simulink model "check_Transmission"  (R2018b)
settings: configuration reference "Physics" (kept outside this file)
model workspace (MAT data in the model file):
  veh_param = Simulink.Parameter
  veh_param.Value.cLiftF = 0
  veh_param.Value.cLiftR = 0
  veh_param.Value.CoGx_m = 0
  veh_param.Value.CoGy_m = 0
  veh_param.Value.CoGz_m = 0
  veh_param.Value.cDrag = 0
  veh_param.Value.Aref_m2 = 0
  veh_param.Value.Gearratio = 0
  veh_param.Value.Wheelbase_m = 0
  veh_param.Value.PacLatF = [0 0 0 0 0]
  veh_param.Value.PacLongF = [0 0 0 0 0]
  veh_param.Value.PacLatR = [0 0 0 0 0]
  veh_param.Value.PacLongR = [0 0 0 0 0]
  veh_param.Value.cRollFriction_Npmps = 0
  veh_param.Value.MaxRollFriction_N = 0
  veh_param.Value.T_YawRate_s = 0
  veh_param.Value.T_LatVel_s = 0
  veh_param.Value.TrackWidthF_m = 0
  veh_param.Value.TrackWidthR_m = 0
  veh_param.Value.TireRadiusF_m = 0
  veh_param.Value.TireRadiusR_m = 0
  veh_param.Value.VehicleInertia_kgm2 = 0
  veh_param.Value.WheelInertiaF_kgm2 = 0
  veh_param.Value.WheelInertiaR_kgm2 = 0
  veh_param.Value.VehicleMass_kg = 0
  veh_param.Value.switchModelBlend_mps = 0
  veh_param.Value.PTLimitLowVel_N = 0
  veh_param.Value.switchModelVel_mps = 0
  veh_param.Value.T_Tire_s = 0
  veh_param.DataType = 'struct'
  veh_param.Dimensions = [1 1]
  x0_positionstates = Simulink.Parameter
  x0_positionstates.Value = [0 0 0]
  x0_positionstates.DataType = 'auto'
  x0_positionstates.Dimensions = [1 3]
undefined symbols (not defined in the file): POWTR__ENGINE__n_lb_rpm__1, POWTR__ENGINE__n_lb_rpm__2, POWTR__ENGINE__n_lb_rpm__3, POWTR__ENGINE__n_lb_rpm__4, POWTR__ENGINE__n_lb_rpm__5, POWTR__ENGINE__n_lb_rpm__6, POWTR__ENGINE__n_lb_rpm__7, POWTR__TRANSMISSION__gear__1, POWTR__TRANSMISSION__gear__2, POWTR__TRANSMISSION__gear__3, POWTR__TRANSMISSION__gear__4, POWTR__TRANSMISSION__gear__5, POWTR__TRANSMISSION__gear__6, POWTR__TRANSMISSION__gear__7, POWTR__TRANSMISSION__gear_efficiency__1, POWTR__TRANSMISSION__gear_efficiency__2, POWTR__TRANSMISSION__gear_efficiency__3, POWTR__TRANSMISSION__gear_efficiency__4, POWTR__TRANSMISSION__gear_efficiency__5, POWTR__TRANSMISSION__gear_efficiency__6, POWTR__TRANSMISSION__gear_efficiency__7, POWTR__TRANSMISSION__gear_ratio__1, POWTR__TRANSMISSION__gear_ratio__2, POWTR__TRANSMISSION__gear_ratio__3, POWTR__TRANSMISSION__gear_ratio__4, POWTR__TRANSMISSION__gear_ratio__5, POWTR__TRANSMISSION__gear_ratio__6, POWTR__TRANSMISSION__gear_ratio__7
settings Model: DataDictionary=vehicleparameters_vehdynsim.sldd  OrderedModelArguments=off  Creator=wischnewski  LastModifiedBy=ga25xiw

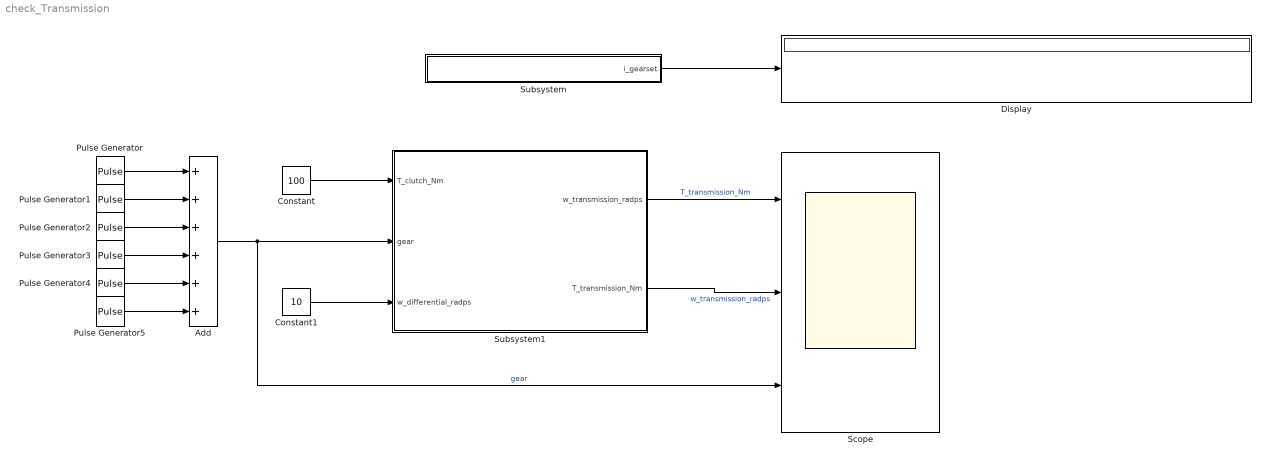
== system check_Transmission ==
  Add : Sum  Inputs=++++++
  Constant : Constant  Value=100
  Constant1 : Constant  Value=10
  Display : Display
  Pulse Generator : DiscretePulseGenerator  PulseType=Time based  Period=10  PulseWidth=90  PhaseDelay=2
  Pulse Generator1 : DiscretePulseGenerator  PulseType=Time based  Period=10  PulseWidth=90  PhaseDelay=3
  Pulse Generator2 : DiscretePulseGenerator  PulseType=Time based  Period=10  PulseWidth=90  PhaseDelay=4
  Pulse Generator3 : DiscretePulseGenerator  PulseType=Time based  Period=10  PulseWidth=90  PhaseDelay=5
  Pulse Generator4 : DiscretePulseGenerator  PulseType=Time based  Period=10  PulseWidth=90  PhaseDelay=6
  Pulse Generator5 : DiscretePulseGenerator  PulseType=Time based  Period=10  PulseWidth=90  PhaseDelay=7
  Scope : Scope  NumInputPorts=3
  Subsystem : Subsystem
  Subsystem1 : Subsystem
  wires:
  Subsystem1/1(w_transmission_radps) -> Scope/1  "T_transmission_Nm"
  Subsystem1/2(T_transmission_Nm) -> Scope/2  "w_transmission_radps"
  Constant/1 -> Subsystem1/1(T_clutch_Nm)
  Pulse Generator/1 -> Add/1
  Pulse Generator1/1 -> Add/2
  Pulse Generator2/1 -> Add/3
  Pulse Generator3/1 -> Add/4
  Pulse Generator4/1 -> Add/5
  Pulse Generator5/1 -> Add/6
  Add/1 -> Subsystem1/2(gear), Scope/3  "gear"
  Constant1/1 -> Subsystem1/3(w_differential_radps)
  Subsystem/1(i_gearset) -> Display/1

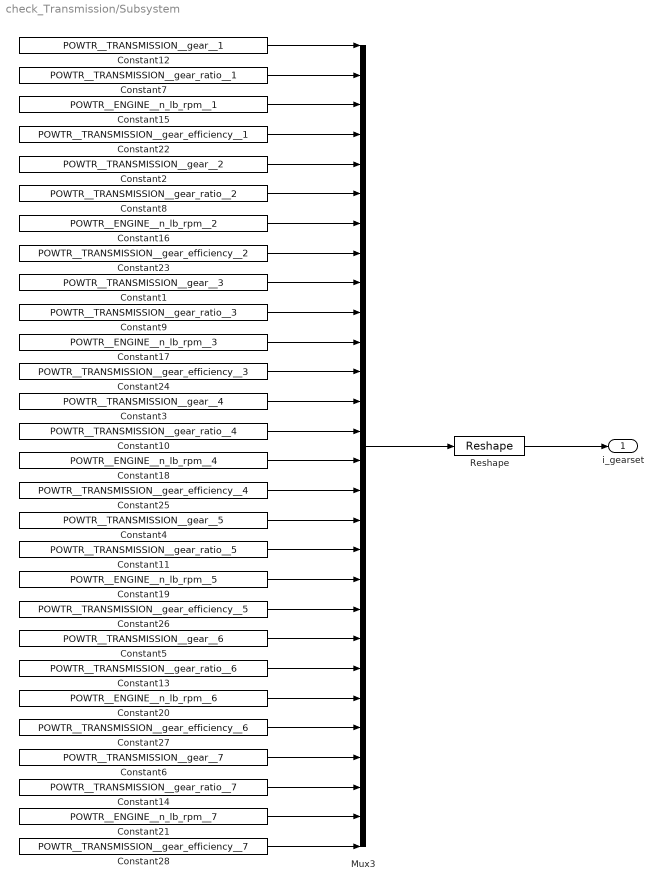
== system check_Transmission/Subsystem ==
  Constant1 : Constant  Value=POWTR__TRANSMISSION__gear__3
  Constant10 : Constant  Value=POWTR__TRANSMISSION__gear_ratio__4
  Constant11 : Constant  Value=POWTR__TRANSMISSION__gear_ratio__5
  Constant12 : Constant  Value=POWTR__TRANSMISSION__gear__1
  Constant13 : Constant  Value=POWTR__TRANSMISSION__gear_ratio__6
  Constant14 : Constant  Value=POWTR__TRANSMISSION__gear_ratio__7
  Constant15 : Constant  Value=POWTR__ENGINE__n_lb_rpm__1
  Constant16 : Constant  Value=POWTR__ENGINE__n_lb_rpm__2
  Constant17 : Constant  Value=POWTR__ENGINE__n_lb_rpm__3
  Constant18 : Constant  Value=POWTR__ENGINE__n_lb_rpm__4
  Constant19 : Constant  Value=POWTR__ENGINE__n_lb_rpm__5
  Constant2 : Constant  Value=POWTR__TRANSMISSION__gear__2
  Constant20 : Constant  Value=POWTR__ENGINE__n_lb_rpm__6
  Constant21 : Constant  Value=POWTR__ENGINE__n_lb_rpm__7
  Constant22 : Constant  Value=POWTR__TRANSMISSION__gear_efficiency__1
  Constant23 : Constant  Value=POWTR__TRANSMISSION__gear_efficiency__2
  Constant24 : Constant  Value=POWTR__TRANSMISSION__gear_efficiency__3
  Constant25 : Constant  Value=POWTR__TRANSMISSION__gear_efficiency__4
  Constant26 : Constant  Value=POWTR__TRANSMISSION__gear_efficiency__5
  Constant27 : Constant  Value=POWTR__TRANSMISSION__gear_efficiency__6
  Constant28 : Constant  Value=POWTR__TRANSMISSION__gear_efficiency__7
  Constant3 : Constant  Value=POWTR__TRANSMISSION__gear__4
  Constant4 : Constant  Value=POWTR__TRANSMISSION__gear__5
  Constant5 : Constant  Value=POWTR__TRANSMISSION__gear__6
  Constant6 : Constant  Value=POWTR__TRANSMISSION__gear__7
  Constant7 : Constant  Value=POWTR__TRANSMISSION__gear_ratio__1
  Constant8 : Constant  Value=POWTR__TRANSMISSION__gear_ratio__2
  Constant9 : Constant  Value=POWTR__TRANSMISSION__gear_ratio__3
  Mux3 : Mux  Inputs=28
  Reshape : Reshape  OutputDimensionality=Customize  OutputDimensions=[4,7]
  i_gearset : Outport
  wires:
  Mux3/1 -> Reshape/1
  Constant12/1 -> Mux3/1
  Reshape/1 -> i_gearset/1
  Constant2/1 -> Mux3/5
  Constant1/1 -> Mux3/9
  Constant3/1 -> Mux3/13
  Constant4/1 -> Mux3/17
  Constant5/1 -> Mux3/21
  Constant6/1 -> Mux3/25
  Constant7/1 -> Mux3/2
  Constant8/1 -> Mux3/6
  Constant9/1 -> Mux3/10
  Constant10/1 -> Mux3/14
  Constant11/1 -> Mux3/18
  Constant13/1 -> Mux3/22
  Constant14/1 -> Mux3/26
  Constant15/1 -> Mux3/3
  Constant16/1 -> Mux3/7
  Constant17/1 -> Mux3/11
  Constant18/1 -> Mux3/15
  Constant19/1 -> Mux3/19
  Constant20/1 -> Mux3/23
  Constant21/1 -> Mux3/27
  Constant22/1 -> Mux3/4
  Constant23/1 -> Mux3/8
  Constant24/1 -> Mux3/12
  Constant25/1 -> Mux3/16
  Constant26/1 -> Mux3/20
  Constant27/1 -> Mux3/24
  Constant28/1 -> Mux3/28

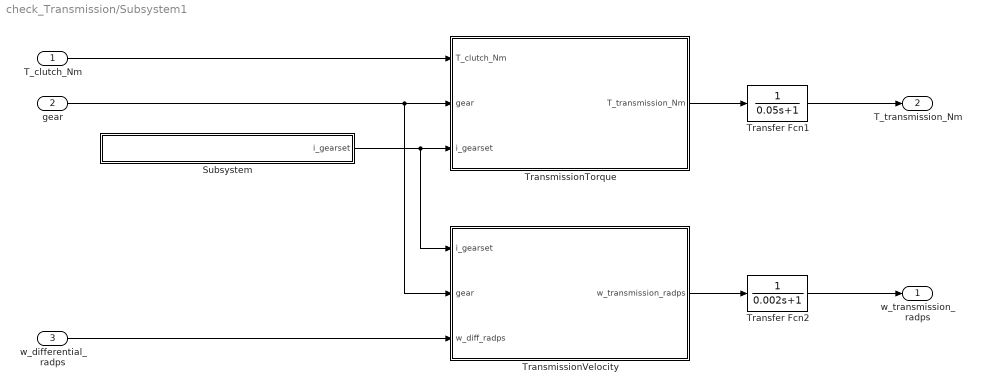
== system check_Transmission/Subsystem1 ==
  T_clutch_Nm : Inport
  gear : Inport  Port=2
  w_differential_radps : Inport  Port=3
  Subsystem : Subsystem
  Transfer Fcn1 : TransferFcn  Denominator=[0.05 1]
  Transfer Fcn2 : TransferFcn  Denominator=[0.002 1]
  TransmissionTorque : MATLAB Function  TreatAsAtomicUnit=on
  TransmissionVelocity : MATLAB Function  TreatAsAtomicUnit=on
  w_transmission_radps : Outport
  T_transmission_Nm : Outport  Port=2
  wires:
  Transfer Fcn1/1 -> T_transmission_Nm/1
  gear/1 -> TransmissionTorque/2(gear), TransmissionVelocity/2(gear)
  Subsystem/1(i_gearset) -> TransmissionTorque/3(i_gearset), TransmissionVelocity/1(i_gearset)
  w_differential_radps/1 -> TransmissionVelocity/3(w_diff_radps)
  Transfer Fcn2/1 -> w_transmission_radps/1
  T_clutch_Nm/1 -> TransmissionTorque/1(T_clutch_Nm)
  TransmissionVelocity/1(w_transmission_radps) -> Transfer Fcn2/1
  TransmissionTorque/1(T_transmission_Nm) -> Transfer Fcn1/1

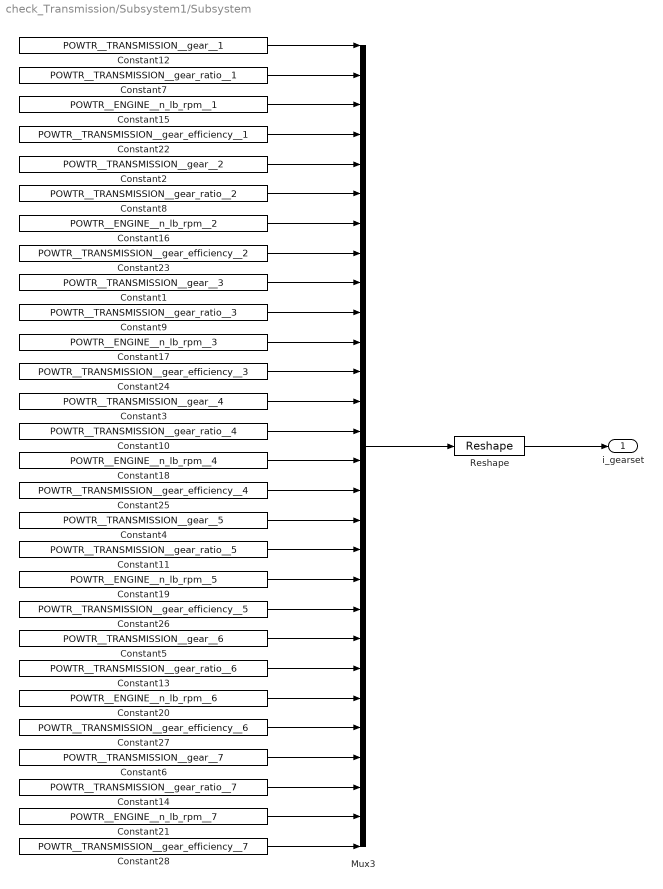
== system check_Transmission/Subsystem1/Subsystem ==
  Constant1 : Constant  Value=POWTR__TRANSMISSION__gear__3
  Constant10 : Constant  Value=POWTR__TRANSMISSION__gear_ratio__4
  Constant11 : Constant  Value=POWTR__TRANSMISSION__gear_ratio__5
  Constant12 : Constant  Value=POWTR__TRANSMISSION__gear__1
  Constant13 : Constant  Value=POWTR__TRANSMISSION__gear_ratio__6
  Constant14 : Constant  Value=POWTR__TRANSMISSION__gear_ratio__7
  Constant15 : Constant  Value=POWTR__ENGINE__n_lb_rpm__1
  Constant16 : Constant  Value=POWTR__ENGINE__n_lb_rpm__2
  Constant17 : Constant  Value=POWTR__ENGINE__n_lb_rpm__3
  Constant18 : Constant  Value=POWTR__ENGINE__n_lb_rpm__4
  Constant19 : Constant  Value=POWTR__ENGINE__n_lb_rpm__5
  Constant2 : Constant  Value=POWTR__TRANSMISSION__gear__2
  Constant20 : Constant  Value=POWTR__ENGINE__n_lb_rpm__6
  Constant21 : Constant  Value=POWTR__ENGINE__n_lb_rpm__7
  Constant22 : Constant  Value=POWTR__TRANSMISSION__gear_efficiency__1
  Constant23 : Constant  Value=POWTR__TRANSMISSION__gear_efficiency__2
  Constant24 : Constant  Value=POWTR__TRANSMISSION__gear_efficiency__3
  Constant25 : Constant  Value=POWTR__TRANSMISSION__gear_efficiency__4
  Constant26 : Constant  Value=POWTR__TRANSMISSION__gear_efficiency__5
  Constant27 : Constant  Value=POWTR__TRANSMISSION__gear_efficiency__6
  Constant28 : Constant  Value=POWTR__TRANSMISSION__gear_efficiency__7
  Constant3 : Constant  Value=POWTR__TRANSMISSION__gear__4
  Constant4 : Constant  Value=POWTR__TRANSMISSION__gear__5
  Constant5 : Constant  Value=POWTR__TRANSMISSION__gear__6
  Constant6 : Constant  Value=POWTR__TRANSMISSION__gear__7
  Constant7 : Constant  Value=POWTR__TRANSMISSION__gear_ratio__1
  Constant8 : Constant  Value=POWTR__TRANSMISSION__gear_ratio__2
  Constant9 : Constant  Value=POWTR__TRANSMISSION__gear_ratio__3
  Mux3 : Mux  Inputs=28
  Reshape : Reshape  OutputDimensionality=Customize  OutputDimensions=[4,7]
  i_gearset : Outport
  wires:
  Mux3/1 -> Reshape/1
  Constant12/1 -> Mux3/1
  Reshape/1 -> i_gearset/1
  Constant2/1 -> Mux3/5
  Constant1/1 -> Mux3/9
  Constant3/1 -> Mux3/13
  Constant4/1 -> Mux3/17
  Constant5/1 -> Mux3/21
  Constant6/1 -> Mux3/25
  Constant7/1 -> Mux3/2
  Constant8/1 -> Mux3/6
  Constant9/1 -> Mux3/10
  Constant10/1 -> Mux3/14
  Constant11/1 -> Mux3/18
  Constant13/1 -> Mux3/22
  Constant14/1 -> Mux3/26
  Constant15/1 -> Mux3/3
  Constant16/1 -> Mux3/7
  Constant17/1 -> Mux3/11
  Constant18/1 -> Mux3/15
  Constant19/1 -> Mux3/19
  Constant20/1 -> Mux3/23
  Constant21/1 -> Mux3/27
  Constant22/1 -> Mux3/4
  Constant23/1 -> Mux3/8
  Constant24/1 -> Mux3/12
  Constant25/1 -> Mux3/16
  Constant26/1 -> Mux3/20
  Constant27/1 -> Mux3/24
  Constant28/1 -> Mux3/28

== matlab function check_Transmission/Subsystem1/TransmissionTorque ==
  data: T_clutch_Nm input; gear input; T_transmission_Nm output; i_gearset input
function T_transmission_Nm = fcn(T_clutch_Nm, gear, i_gearset)

T_transmission_Nm = TransmissionTorque(T_clutch_Nm, gear, i_gearset);

== matlab function check_Transmission/Subsystem1/TransmissionVelocity ==
  data: i_gearset input; w_transmission_radps output; gear input; w_diff_radps input
function w_transmission_radps = fcn(i_gearset, gear, w_diff_radps)

w_transmission_radps = TransmissionVelocity(i_gearset, gear, w_diff_radps);
